simulink model "full_model"  (R2015b)
settings: Solver=FixedStepAuto  StartTime=0.0  StopTime=30  FixedStep=Ts  MaxStep=0.005  RelTol=1e-3
InitFcn:
  | Ts=0.01;
values from neighbouring files (symbols this model uses):
  A = [-1/Tg1     0      -1/(R1*Tg1)   0       0       0        0 ... (first row only)    [fullModel_2area.m]
  B = [ 1/Tg1 0    0    0 ... (first row only)    [fullModel_2area.m]
  C = [0 0 B1  1 0 0 0 ... (first row only)    [fullModel_2area.m]
  dPL1 = 1    [fullModel_2area.m]
  dPL2 = 0    [fullModel_2area.m]
settings Model: Creator=Majidi  LastModifiedBy=Admin
settings DataIOCC: SaveFormat=Array
settings OptimizationCC: ExpressionDepthLimit=2147483647
settings DebuggingCC: UnderspecifiedInitializationDetection=Classic  MergeDetectMultiDrivingBlocksExec=none  SolverPrmCheckMsg=warning  StateNameClashWarn=warning
settings HardwareCC: ProdBitPerPointer=32  ProdLargestAtomicFloat=None  ProdIntDivRoundTo=Undefined  ProdEndianess=Unspecified  ProdWordSize=32  ProdHWDeviceType=32-bit Generic
settings GRTTargetCC: GeneratePreprocessorConditionals=Disable all
settings ConfigComp: CovModelRefEnable=Off

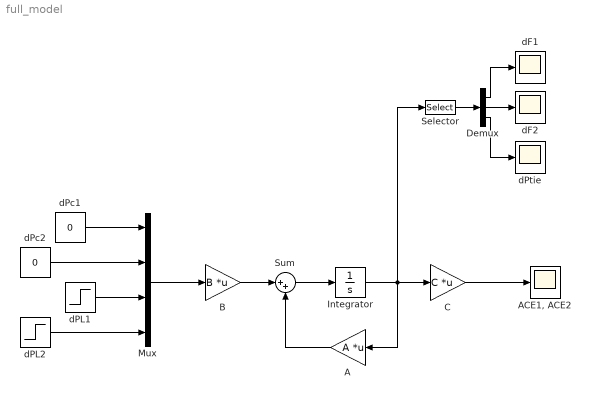
== system full_model ==
  A : Gain  Gain=A  Multiplication=Matrix(K*u)
  "ACE1, ACE2" : Scope
  B : Gain  Gain=B  Multiplication=Matrix(K*u)
  C : Gain  Gain=C  Multiplication=Matrix(K*u)
  Demux : Demux  Outputs=3
  Integrator : Integrator
  Mux : Mux
  Selector : Selector  InputPortWidth=7  IndexOptions=Index vector (dialog)  Indices=[3 4 7]  OutputSizes=1
  Sum : Sum  Inputs=|++
  dF1 : Scope
  dF2 : Scope
  dPL1 : Step  After=dPL1  SampleTime=0
  dPL2 : Step  After=dPL2  SampleTime=0
  dPc1 : Constant  Value=0
  dPc2 : Constant  Value=0
  dPtie : Scope
  wires:
  B/1 -> Sum/1
  Sum/1 -> Integrator/1
  A/1 -> Sum/2
  Integrator/1 -> Selector/1, A/1, C/1
  C/1 -> "ACE1, ACE2"/1
  Mux/1 -> B/1
  dPL1/1 -> Mux/3
  dPL2/1 -> Mux/4
  dPc1/1 -> Mux/1
  dPc2/1 -> Mux/2
  Demux/1 -> dF1/1
  Demux/2 -> dF2/1
  Demux/3 -> dPtie/1
  Selector/1 -> Demux/1
